simulink model "V2GStronge2_published_controller"  (R2024a)
settings: Solver=odeN  StartTime=0.0  StopTime=36000  FixedStep=10
model workspace (MAT data in the model file):
  Soc = 75
undefined symbols (not defined in the file): Ion, Lithium
libraries: spsMosfetLib x14, spsSeriesRLCBranchLib x14, slpidlib x8, spsBatteryLib x4, spsPWMGeneratorDCDCLib x4, spsCurrentMeasurementLib x3, spsAlphaBetaZerotodq0Lib x2, spsGroundLib x1, spsPWMGenerator2LevelLib x1, eePowerMeasurement x1, spsThreePhaseVIMeasurementLib x1, spsThreePhaseSourceLib x1
(part 1 of 2)
settings Model: SimulationMode=accelerator  PacingRate=1000  VariantFading=off  Creator=Mahmoud Kiasari  LastModifiedBy=mtk17
settings SolverCC: ZeroCrossControl=DisableAll  ZeroCrossAlgorithm=Adaptive  ODENIntegrationMethod=ode1
settings DataIOCC: ExternalInput=HouseHoldConsumption  SaveOutput=off  SignalLogging=off  DSMLogging=off  SaveTime=off  ReturnWorkspaceOutputs=off  OutputOption=SpecifiedOutputTimes  OutputTimes=OutTime
settings OptimizationCC: DefaultUnderspecifiedDataType=single  ReuseModelBlockBuffer=off
settings DebuggingCC: IgnoredZcDiagnostic=none  UnconnectedInputMsg=warning  UnconnectedOutputMsg=warning  UnconnectedLineMsg=warning
settings ModelReferenceCC: UpdateModelReferenceTargets=AssumeUpToDate  CheckModelReferenceTargetMessage=warning  EnableParallelModelReferenceBuilds=on  ModelReferenceNumInstancesAllowed=Zero  PropagateSignalLabelsOutOfModel=off
settings SFSimCC: SimTargetLang=C++  GPUAcceleration=on  SimDLTargetLibrary=cudnn
settings RTWCC: GPUComputeCapability=3.5  DLArmComputeVersion=19.05

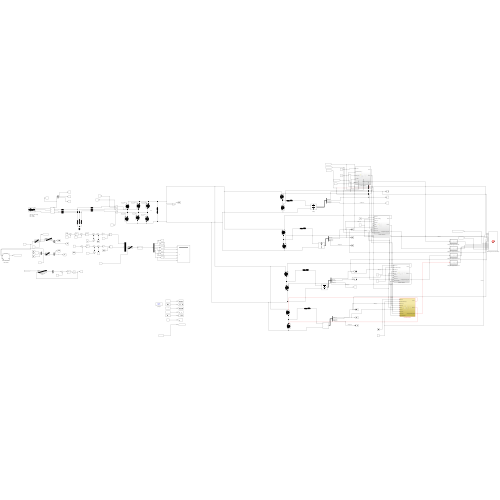
[thumbnail: Simulink's stored preview of the top-level diagram]
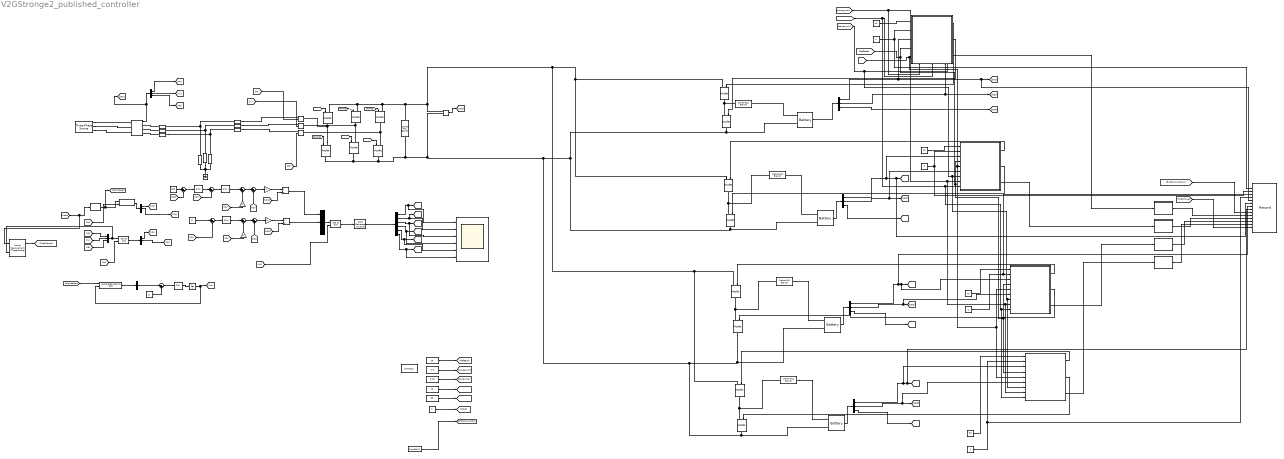
== system V2GStronge2_published_controller ==
  note: Battery
  note: Vdc
  note: 208V line to line voltage
      | Fsw = 10Khz
      | Fres = 1000hz
  Alpha-Beta-Zero to dq0 : spsAlphaBetaZerotodq0Lib/Alpha-Beta-Zero to dq0  Alignment=90 degrees behind phase A axis
  Alpha-Beta-Zero to dq1 : spsAlphaBetaZerotodq0Lib/Alpha-Beta-Zero to dq0  Alignment=90 degrees behind phase A axis
  Battery : spsBatteryLib/Battery  BatType=Lithium-Ion  ShowTempParam=off  ThermalPreset=no  ShowAgeParam=off  NomV=360  NomQ=62  SOC=90  Batt_Tr=1  PresetModel=off  MaxQ=300  MinV=270  FullV=419.0354  Dis_rate=130.4348  R=0.012  Normal_OP=271.3043  expZone="[388.9389      14.73913]"  current=[6.5 13 32.5]  Units=Time  Tci=20  NomT=20  T2=0  MaxQ2=300  FullV2=300  Normal_OP2=270  expZone2="[388.9389      14.73913]"  Rca=0.6411  ti=4880  Dp=0  Neq0=0  Tsim=1e6  Ta1=25  Qeol=5.4*0.9  Reol=0.013333*1.2  Char_age=[2.3478, 3]  Dis_age=[2.3478, 10]  N1=1500  N2=10500  N3=1000  N4=1400  Ta2=45  N5=950
  Battery1 : spsBatteryLib/Battery  BatType=Lithium-Ion  ShowTempParam=off  ThermalPreset=no  ShowAgeParam=off  NomV=375  NomQ=100  SOC=70  Batt_Tr=1  PresetModel=on  MaxQ=100  MinV=281.25  FullV=436.4952  Dis_rate=43.4783  R=0.0375  Normal_OP=90.4348  expZone="[405.1447      4.913043]"  current=[6.5 13 32.5]  Units=Time  Tci=20  NomT=20  T2=0  MaxQ2=300  FullV2=300  Normal_OP2=270  expZone2="[388.9389      14.73913]"  Rca=0.6411  ti=4880  Dp=0  Neq0=0  Tsim=1e6  Ta1=25  Qeol=5.4*0.9  Reol=0.013333*1.2  Char_age=[2.3478, 3]  Dis_age=[2.3478, 10]  N1=1500  N2=10500  N3=1000  N4=1400  Ta2=45  N5=950
  Battery2 : spsBatteryLib/Battery  BatType=Lithium-Ion  ShowTempParam=off  ThermalPreset=no  ShowAgeParam=off  NomV=360  NomQ=94  SOC=50  Batt_Tr=1  PresetModel=off  MaxQ=300  MinV=270  FullV=419.0354  Dis_rate=130.4348  R=0.012  Normal_OP=271.3043  expZone="[388.9389      14.73913]"  current=[6.5 13 32.5]  Units=Ampere-hour  Tci=20  NomT=20  T2=0  MaxQ2=300  FullV2=300  Normal_OP2=270  expZone2="[388.9389      14.73913]"  Rca=0.6411  ti=4880  Dp=0  Neq0=0  Tsim=1e6  Ta1=25  Qeol=5.4*0.9  Reol=0.013333*1.2  Char_age=[2.3478, 3]  Dis_age=[2.3478, 10]  N1=1500  N2=10500  N3=1000  N4=1400  Ta2=45  N5=950
  Battery3 : spsBatteryLib/Battery  BatType=Lithium-Ion  ShowTempParam=off  ThermalPreset=no  ShowAgeParam=off  NomV=396  NomQ=95  SOC=30  Batt_Tr=1  PresetModel=on  MaxQ=95  MinV=297  FullV=460.9389  Dis_rate=41.3043  R=0.041684  Normal_OP=85.913  expZone="[427.8328      4.667391]"  current=[6.5 13 32.5]  Units=Time  Tci=20  NomT=20  T2=0  MaxQ2=300  FullV2=300  Normal_OP2=270  expZone2="[388.9389      14.73913]"  Rca=0.6411  ti=4880  Dp=0  Neq0=0  Tsim=1e6  Ta1=25  Qeol=5.4*0.9  Reol=0.013333*1.2  Char_age=[2.3478, 3]  Dis_age=[2.3478, 10]  N1=1500  N2=10500  N3=1000  N4=1400  Ta2=45  N5=950
  Bus Selector{,1..3} (4 alike) : BusSelector  OutputSignals=SOC (%),Current (A),Voltage (V)
  Charge/Discharge/Ideal Detection : Subsystem  TreatAsAtomicUnit=on
  Charge/Discharge/Ideal Detection1 : Subsystem  TreatAsAtomicUnit=on
  Charge/Discharge/Ideal Detection2 : Subsystem  TreatAsAtomicUnit=on
  Charge/Discharge/Ideal Detection3 : Subsystem  TreatAsAtomicUnit=on
  Condition checker 1 : Subsystem
      settings: PortSchema="{\"entries\":[{\"content\":{\"sides\":[{\"content\":{\"connectorIds\":[\"In1\",\"In2\",\"In3\",\"In4\",\"In5\"]},\"type\":\"ConnectorPlacement.EquallySpacedRectSide\",\"uuid\":\"c002707d-8367-4a40-a9c2-601c499a357e\"},{\"content\":{\"connectorIds\":[\"Out1\",\"Out2\",\"Out3\"],\"side\":\"RIGHT\"},\"type\":\"ConnectorPlacement.EquallySpacedRectSide\",\"uuid\":\"668af4fe-86d6-4dea-905e-b454fc1f82cc\"},{\"content\":{\"side\":\"TOP\"},\"type\":\"ConnectorPlacement.EquallySpacedRectSide\",\"uuid\":\"2ab59da3-7144-4706-b30d-a458153a4ce4\"},{\"content\":{\"connectorIds\":[\"In6\",\"In7\",\"In8\"],\"side\":\"BOTTOM\"},\"type\":\"ConnectorPlacement.EquallySpacedRectSide\",\"uuid\":\"16d703a8-fda5-4631-9c2f-f2e45db3531f\"}]},\"type\":\"ConnectorPlacement.EquallySpacedConnector\",\"uuid\":\"736966d1-dbcb-4619-a26f-9e7ed5309763\"}],\"packageUris\":[\"http://schema.mathworks.com/mf0/Connector/R2020b\"],\"version\":\"1.0\"}"
  Condition checker 2 : Subsystem
  Condition checker 3 : Subsystem
  Condition checker 4 : Subsystem
  Constant : Constant  Value=0
  Constant1 : Constant  Value=400
  Constant10 : Constant  SampleTime=0
  Constant{6,9,12..13} (4 alike) : Constant  Value=40  SampleTime=0
  Constant14 : Constant  Value=-1  SampleTime=0
  Constant15 : Constant  Value=50  SampleTime=0
  Constant16 : Constant  SampleTime=0
  Constant17 : Constant  SampleTime=0
  Constant2 : Constant  Value=0
  Constant3 : Constant  Value=20  SampleTime=0
  Constant4 : Constant  Value=2.9  SampleTime=0
  Constant5 : Constant  Value=9.25  SampleTime=0
  Constant7 : Constant  Value=60  SampleTime=0
  Constant8 : Constant  Value=0  SampleTime=0
  Current Measurement : spsCurrentMeasurementLib/Current Measurement  PhasorSimulation=off  OutputType=Complex  PSBequivalent=0
  Current Measurement1 : spsCurrentMeasurementLib/Current Measurement  PhasorSimulation=off  OutputType=Complex  PSBequivalent=0
  Current Measurement2 : spsCurrentMeasurementLib/Current Measurement  PhasorSimulation=off  OutputType=Complex  PSBequivalent=0
  Demux{,1..2,4} (4 alike) : Demux  Outputs=3
  Demux3 : Demux  Outputs=6
  From Workspace : FromWorkspace  VariableName=from3to12  SampleTime=60
  Gain : Gain  Gain=2*3.14*60*10e-3
  Gain1 : Gain  Gain=2
  Gain2 : Gain  Gain=2*3.14*60*10e-3
  Gain3 : Gain  Gain=2
  Ground2 : spsGroundLib/Ground  LConnTagsString=a
  Integrator : Integrator
  Mosfet{,1,3..14} (14 alike) : spsMosfetLib/Mosfet  Ron=0.1  Lon=0  Rd=0.01  Vfd=0  IC=0  Rs=1e5  Cs=inf  Measurements=off
  Mux : Mux  Inputs=3
  Mux1 : Mux  Inputs=3
  PID Controller : slpidlib/PID Controller  Controller=PI  Form=Parallel  TimeDomain=Discrete-time  UseExternalTs=off  SampleTime=-1  IntegratorMethod=Forward Euler  FilterMethod=Forward Euler  ControllerParametersSource=internal  P=10  I=50000  UseKiTs=off  D=0  UseExternalDerivativeSource=off  N=100  UseFilter=on  TunerSelectOption=Transfer Function Based (PID Tuner App)  InitialConditionSource=internal  InitialConditionForIntegrator=0  InitialConditionForFilter=0  DifferentiatorICPrevScaledInput=0  ExternalReset=none  TrackingMode=off  Kt=1  LimitOutput=off  SatLimitsSource=internal  UpperSaturationLimit=0.95  LowerSaturationLimit=0  LinearizeAsGain=on  AntiWindupMode=none  Kb=1  LimitIntegrator=off  UpperIntegratorSaturationLimit=inf  LowerIntegratorSaturationLimit=-inf  POutMin=[]  POutMax=[]  IOutMin=[]  IOutMax=[]  DOutMin=[]  DOutMax=[]  NOutMin=[]  NOutMax=[]  SumOutMin=[]  SumOutMax=[]  SaturationOutMin=[]  SaturationOutMax=[]  PParamMin=[]  PParamMax=[]  IParamMin=[]  IParamMax=[]  DParamMin=[]  DParamMax=[]  NParamMin=[]  NParamMax=[]  KbParamMin=[]  KbParamMax=[]  KtParamMin=[]  KtParamMax=[]  KbOutMin=[]  KbOutMax=[]  KtOutMin=[]  KtOutMax=[]  IntegratorOutMin=[]  IntegratorOutMax=[]  FilterOutMin=[]  FilterOutMax=[]  SumI1OutMin=[]  SumI1OutMax=[]  SumI2OutMin=[]  SumI2OutMax=[]  SumI3OutMin=[]  SumI3OutMax=[]  SumI4OutMin=[]  SumI4OutMax=[]  SumDOutMin=[]  SumDOutMax=[]  DifferentiatorOutMin=[]  DifferentiatorOutMax=[]  FilterDiffOutCoefMin=[]  FilterDiffOutCoefMax=[]  ReciprocalOutMin=[]  ReciprocalOutMax=[]  SumDenOutMin=[]  SumDenOutMax=[]  SumNumOutMin=[]  SumNumOutMax=[]  DivideOutMin=[]  DivideOutMax=[]  UdiffTsProdOutMin=[]  UdiffTsProdOutMax=[]  NTsProdOutMin=[]  NTsProdOutMax=[]  UintegralTsProdOutMin=[]  UintegralTsProdOutMax=[]  UngainTsProdOutMin=[]  UngainTsProdOutMax=[]  ClampingZeroOutDataTypeStr=Inherit: Inherit via back propagation  ClampingZeroOutMin=[]  ClampingZeroOutMax=[]  FilterDenConstantOutDataTypeStr=Inherit: Inherit via back propagation  FilterDenConstantOutMin=[]  FilterDenConstantOutMax=[]  PCopyOutDataTypeStr=Inherit: Inherit via back propagation  PCopyOutMin=[]  PCopyOutMax=[]  NCopyOutDataTypeStr=Inherit: Inherit via back propagation  NCopyOutMin=[]  NCopyOutMax=[]  IntegratorContinuousStateAttributes=''  IntegratorStateMustResolveToSignalObject=off  IntegratorRTWStateStorageClass=Auto  FilterContinuousStateAttributes=''  FilterStateMustResolveToSignalObject=off  FilterRTWStateStorageClass=Auto  ParallelPVariant=InternalParameters  IdealPVariant=Disabled  IVariant=InternalParameters  DVariant=Disabled  IntegratorVariant=Discrete  SatVariant=Disabled  AWVariant=Passthrough  PCopyVariant=Disabled  TRVariant=Disabled  FdbkBlocksVariant=Forward  IdealPFdbkVariant=Disabled  SatFdbkVariant=Disabled  DerivativeFilterVariant=Disabled  NVariant=Disabled  NCopyVariant=Disabled_SignalSpec  FilterICVariant=Disabled  IntegratorICVariant=InternalICs  ExternalResetVariant=Disabled  TRSumVariant=Passthrough  SumFdbkVariant=Disabled  SumVariant=Sum_PI  TsampFilterVariant=InternalTs  TsampNgainVariant=Passthrough  TsampIntegralVariant=Disabled_SignalSpec  ExternalSaturationOutDataTypeStr=Inherit: Same as second input  DerivativeSourceVariant=Disabled
  PID Controller1 : slpidlib/PID Controller  Controller=PI  Form=Parallel  TimeDomain=Continuous-time  UseExternalTs=off  SampleTime=-1  IntegratorMethod=Forward Euler  FilterMethod=Forward Euler  ControllerParametersSource=internal  P=0.5  I=5  UseKiTs=off  D=0  UseExternalDerivativeSource=off  N=100  UseFilter=on  TunerSelectOption=Transfer Function Based (PID Tuner App)  InitialConditionSource=internal  InitialConditionForIntegrator=0  InitialConditionForFilter=0  DifferentiatorICPrevScaledInput=0  ExternalReset=none  TrackingMode=off  Kt=1  LimitOutput=off  SatLimitsSource=internal  UpperSaturationLimit=inf  LowerSaturationLimit=-inf  LinearizeAsGain=on  AntiWindupMode=none  Kb=1  LimitIntegrator=off  UpperIntegratorSaturationLimit=inf  LowerIntegratorSaturationLimit=-inf  POutMin=[]  POutMax=[]  IOutMin=[]  IOutMax=[]  DOutMin=[]  DOutMax=[]  NOutMin=[]  NOutMax=[]  SumOutMin=[]  SumOutMax=[]  SaturationOutMin=[]  SaturationOutMax=[]  PParamMin=[]  PParamMax=[]  IParamMin=[]  IParamMax=[]  DParamMin=[]  DParamMax=[]  NParamMin=[]  NParamMax=[]  KbParamMin=[]  KbParamMax=[]  KtParamMin=[]  KtParamMax=[]  KbOutMin=[]  KbOutMax=[]  KtOutMin=[]  KtOutMax=[]  IntegratorOutMin=[]  IntegratorOutMax=[]  FilterOutMin=[]  FilterOutMax=[]  SumI1OutMin=[]  SumI1OutMax=[]  SumI2OutMin=[]  SumI2OutMax=[]  SumI3OutMin=[]  SumI3OutMax=[]  SumI4OutMin=[]  SumI4OutMax=[]  SumDOutMin=[]  SumDOutMax=[]  DifferentiatorOutMin=[]  DifferentiatorOutMax=[]  FilterDiffOutCoefMin=[]  FilterDiffOutCoefMax=[]  ReciprocalOutMin=[]  ReciprocalOutMax=[]  SumDenOutMin=[]  SumDenOutMax=[]  SumNumOutMin=[]  SumNumOutMax=[]  DivideOutMin=[]  DivideOutMax=[]  UdiffTsProdOutMin=[]  UdiffTsProdOutMax=[]  NTsProdOutMin=[]  NTsProdOutMax=[]  UintegralTsProdOutMin=[]  UintegralTsProdOutMax=[]  UngainTsProdOutMin=[]  UngainTsProdOutMax=[]  ClampingZeroOutDataTypeStr=Inherit: Inherit via back propagation  ClampingZeroOutMin=[]  ClampingZeroOutMax=[]  FilterDenConstantOutDataTypeStr=Inherit: Inherit via back propagation  FilterDenConstantOutMin=[]  FilterDenConstantOutMax=[]  PCopyOutDataTypeStr=Inherit: Inherit via back propagation  PCopyOutMin=[]  PCopyOutMax=[]  NCopyOutDataTypeStr=Inherit: Inherit via back propagation  NCopyOutMin=[]  NCopyOutMax=[]  IntegratorContinuousStateAttributes=''  IntegratorStateMustResolveToSignalObject=off  IntegratorRTWStateStorageClass=Auto  FilterContinuousStateAttributes=''  FilterStateMustResolveToSignalObject=off  FilterRTWStateStorageClass=Auto  ParallelPVariant=InternalParameters  IdealPVariant=Disabled  IVariant=InternalParameters  DVariant=Disabled  IntegratorVariant=Continuous  SatVariant=Disabled  AWVariant=Passthrough  PCopyVariant=Disabled  TRVariant=Disabled  FdbkBlocksVariant=Forward  IdealPFdbkVariant=Disabled  SatFdbkVariant=Disabled  DerivativeFilterVariant=Disabled  NVariant=Disabled  NCopyVariant=Disabled_SignalSpec  FilterICVariant=Disabled  IntegratorICVariant=InternalICs  ExternalResetVariant=Disabled  TRSumVariant=Passthrough  SumFdbkVariant=Disabled  SumVariant=Sum_PI  TsampFilterVariant=InternalTs  TsampNgainVariant=Passthrough  TsampIntegralVariant=Disabled_SignalSpec  ExternalSaturationOutDataTypeStr=Inherit: Same as second input  DerivativeSourceVariant=Disabled
  PID Controller2 : slpidlib/PID Controller  Controller=PI  Form=Parallel  TimeDomain=Continuous-time  UseExternalTs=off  SampleTime=-1  IntegratorMethod=Forward Euler  FilterMethod=Forward Euler  ControllerParametersSource=internal  P=25  I=500  UseKiTs=off  D=0  UseExternalDerivativeSource=off  N=100  UseFilter=on  TunerSelectOption=Transfer Function Based (PID Tuner App)  InitialConditionSource=internal  InitialConditionForIntegrator=0  InitialConditionForFilter=0  DifferentiatorICPrevScaledInput=0  ExternalReset=none  TrackingMode=off  Kt=1  LimitOutput=off  SatLimitsSource=internal  UpperSaturationLimit=inf  LowerSaturationLimit=-inf  LinearizeAsGain=on  AntiWindupMode=none  Kb=1  LimitIntegrator=off  UpperIntegratorSaturationLimit=inf  LowerIntegratorSaturationLimit=-inf  POutMin=[]  POutMax=[]  IOutMin=[]  IOutMax=[]  DOutMin=[]  DOutMax=[]  NOutMin=[]  NOutMax=[]  SumOutMin=[]  SumOutMax=[]  SaturationOutMin=[]  SaturationOutMax=[]  PParamMin=[]  PParamMax=[]  IParamMin=[]  IParamMax=[]  DParamMin=[]  DParamMax=[]  NParamMin=[]  NParamMax=[]  KbParamMin=[]  KbParamMax=[]  KtParamMin=[]  KtParamMax=[]  KbOutMin=[]  KbOutMax=[]  KtOutMin=[]  KtOutMax=[]  IntegratorOutMin=[]  IntegratorOutMax=[]  FilterOutMin=[]  FilterOutMax=[]  SumI1OutMin=[]  SumI1OutMax=[]  SumI2OutMin=[]  SumI2OutMax=[]  SumI3OutMin=[]  SumI3OutMax=[]  SumI4OutMin=[]  SumI4OutMax=[]  SumDOutMin=[]  SumDOutMax=[]  DifferentiatorOutMin=[]  DifferentiatorOutMax=[]  FilterDiffOutCoefMin=[]  FilterDiffOutCoefMax=[]  ReciprocalOutMin=[]  ReciprocalOutMax=[]  SumDenOutMin=[]  SumDenOutMax=[]  SumNumOutMin=[]  SumNumOutMax=[]  DivideOutMin=[]  DivideOutMax=[]  UdiffTsProdOutMin=[]  UdiffTsProdOutMax=[]  NTsProdOutMin=[]  NTsProdOutMax=[]  UintegralTsProdOutMin=[]  UintegralTsProdOutMax=[]  UngainTsProdOutMin=[]  UngainTsProdOutMax=[]  ClampingZeroOutDataTypeStr=Inherit: Inherit via back propagation  ClampingZeroOutMin=[]  ClampingZeroOutMax=[]  FilterDenConstantOutDataTypeStr=Inherit: Inherit via back propagation  FilterDenConstantOutMin=[]  FilterDenConstantOutMax=[]  PCopyOutDataTypeStr=Inherit: Inherit via back propagation  PCopyOutMin=[]  PCopyOutMax=[]  NCopyOutDataTypeStr=Inherit: Inherit via back propagation  NCopyOutMin=[]  NCopyOutMax=[]  IntegratorContinuousStateAttributes=''  IntegratorStateMustResolveToSignalObject=off  IntegratorRTWStateStorageClass=Auto  FilterContinuousStateAttributes=''  FilterStateMustResolveToSignalObject=off  FilterRTWStateStorageClass=Auto  ParallelPVariant=InternalParameters  IdealPVariant=Disabled  IVariant=InternalParameters  DVariant=Disabled  IntegratorVariant=Continuous  SatVariant=Disabled  AWVariant=Passthrough  PCopyVariant=Disabled  TRVariant=Disabled  FdbkBlocksVariant=Forward  IdealPFdbkVariant=Disabled  SatFdbkVariant=Disabled  DerivativeFilterVariant=Disabled  NVariant=Disabled  NCopyVariant=Disabled_SignalSpec  FilterICVariant=Disabled  IntegratorICVariant=InternalICs  ExternalResetVariant=Disabled  TRSumVariant=Passthrough  SumFdbkVariant=Disabled  SumVariant=Sum_PI  TsampFilterVariant=InternalTs  TsampNgainVariant=Passthrough  TsampIntegralVariant=Disabled_SignalSpec  ExternalSaturationOutDataTypeStr=Inherit: Same as second input  DerivativeSourceVariant=Disabled
  PID Controller3 : slpidlib/PID Controller  Controller=PI  Form=Parallel  TimeDomain=Continuous-time  UseExternalTs=off  SampleTime=-1  IntegratorMethod=Forward Euler  FilterMethod=Forward Euler  ControllerParametersSource=internal  P=25  I=500  UseKiTs=off  D=0  UseExternalDerivativeSource=off  N=100  UseFilter=on  TunerSelectOption=Transfer Function Based (PID Tuner App)  InitialConditionSource=internal  InitialConditionForIntegrator=0  InitialConditionForFilter=0  DifferentiatorICPrevScaledInput=0  ExternalReset=none  TrackingMode=off  Kt=1  LimitOutput=off  SatLimitsSource=internal  UpperSaturationLimit=inf  LowerSaturationLimit=-inf  LinearizeAsGain=on  AntiWindupMode=none  Kb=1  LimitIntegrator=off  UpperIntegratorSaturationLimit=inf  LowerIntegratorSaturationLimit=-inf  POutMin=[]  POutMax=[]  IOutMin=[]  IOutMax=[]  DOutMin=[]  DOutMax=[]  NOutMin=[]  NOutMax=[]  SumOutMin=[]  SumOutMax=[]  SaturationOutMin=[]  SaturationOutMax=[]  PParamMin=[]  PParamMax=[]  IParamMin=[]  IParamMax=[]  DParamMin=[]  DParamMax=[]  NParamMin=[]  NParamMax=[]  KbParamMin=[]  KbParamMax=[]  KtParamMin=[]  KtParamMax=[]  KbOutMin=[]  KbOutMax=[]  KtOutMin=[]  KtOutMax=[]  IntegratorOutMin=[]  IntegratorOutMax=[]  FilterOutMin=[]  FilterOutMax=[]  SumI1OutMin=[]  SumI1OutMax=[]  SumI2OutMin=[]  SumI2OutMax=[]  SumI3OutMin=[]  SumI3OutMax=[]  SumI4OutMin=[]  SumI4OutMax=[]  SumDOutMin=[]  SumDOutMax=[]  DifferentiatorOutMin=[]  DifferentiatorOutMax=[]  FilterDiffOutCoefMin=[]  FilterDiffOutCoefMax=[]  ReciprocalOutMin=[]  ReciprocalOutMax=[]  SumDenOutMin=[]  SumDenOutMax=[]  SumNumOutMin=[]  SumNumOutMax=[]  DivideOutMin=[]  DivideOutMax=[]  UdiffTsProdOutMin=[]  UdiffTsProdOutMax=[]  NTsProdOutMin=[]  NTsProdOutMax=[]  UintegralTsProdOutMin=[]  UintegralTsProdOutMax=[]  UngainTsProdOutMin=[]  UngainTsProdOutMax=[]  ClampingZeroOutDataTypeStr=Inherit: Inherit via back propagation  ClampingZeroOutMin=[]  ClampingZeroOutMax=[]  FilterDenConstantOutDataTypeStr=Inherit: Inherit via back propagation  FilterDenConstantOutMin=[]  FilterDenConstantOutMax=[]  PCopyOutDataTypeStr=Inherit: Inherit via back propagation  PCopyOutMin=[]  PCopyOutMax=[]  NCopyOutDataTypeStr=Inherit: Inherit via back propagation  NCopyOutMin=[]  NCopyOutMax=[]  IntegratorContinuousStateAttributes=''  IntegratorStateMustResolveToSignalObject=off  IntegratorRTWStateStorageClass=Auto  FilterContinuousStateAttributes=''  FilterStateMustResolveToSignalObject=off  FilterRTWStateStorageClass=Auto  ParallelPVariant=InternalParameters  IdealPVariant=Disabled  IVariant=InternalParameters  DVariant=Disabled  IntegratorVariant=Continuous  SatVariant=Disabled  AWVariant=Passthrough  PCopyVariant=Disabled  TRVariant=Disabled  FdbkBlocksVariant=Forward  IdealPFdbkVariant=Disabled  SatFdbkVariant=Disabled  DerivativeFilterVariant=Disabled  NVariant=Disabled  NCopyVariant=Disabled_SignalSpec  FilterICVariant=Disabled  IntegratorICVariant=InternalICs  ExternalResetVariant=Disabled  TRSumVariant=Passthrough  SumFdbkVariant=Disabled  SumVariant=Sum_PI  TsampFilterVariant=InternalTs  TsampNgainVariant=Passthrough  TsampIntegralVariant=Disabled_SignalSpec  ExternalSaturationOutDataTypeStr=Inherit: Same as second input  DerivativeSourceVariant=Disabled
  PWM Generator (2-Level) : spsPWMGenerator2LevelLib/PWM Generator (2-Level)  ModulatorType=Three-phase bridge (6 pulses)  ModulatorMode=Unsynchronized  Fc=60  Pc=90  nF=27  MinMax="[ -1  1 ]"  SamplingTechnique=Natural  ModulatingSignals=off  m=0.8  Freq=60  Phase=0  Ts=0  ShowCarrierOutport=off
  Power Measurement (Three-Phase) : eePowerMeasurement/Power Measurement (Three-Phase)  LabelModeActiveChoice=Continuous  F=60  K=[0 1 2 3]  Seq=Positive  Ts=0
  Product : Product  Inputs=*/
  Product1 : Product  Inputs=*/
  Recording the SoC of each battery : Record  Filename=C:\Users\Mahmoud Kiasari\Desktop\Dalhousie\Thesis\Thesis Versions\Matlab Models\EV V2G and G2V\Data\ThesisData2Hours12to6.xlsx  FileSettingsInternal="{\"entries\":[{\"content\":{\"excelSettings\":{\"content\":{},\"type\":\"Streamout.ExcelSettings\"}},\"type\":\"Streamout.FileSettingStorage\",\"uuid\":\"\"}],\"packageUris\":[\"http:\\/\\/schema.mathworks.com\\/mf0\\/streamout_blocks\\/R2020a\"],\"version\":\"1.0\"}"  Layout=[1 1]  SignalsInternal="{\"entries\":[{\"content\":{\"signals\":[{\"content\":{\"blockPath\":[],\"dimensions\":[1],\"domain\":\"\",\"lineColor\":\"#64d413\",\"port\":1,\"sid\":[\"\"],\"signalID\":1,\"signalName\":\"Owner 1\"},\"type\":\"RecordBlkView.Signal\",\"uuid\":\"\"},{\"content\":{\"blockPath\":[],\"dimensions\":[1],\"domain\":\"\",\"lineColor\":\"#64d413\",\"plots\":[ 9 ],\"port\":2,\"sid\":[\"\"],\"signalID\":2,\"signalName\":\"Owner 2\"},\"type\":\"RecordBlkView.Signal\",\"uuid\":\"\"},{\"content\":{\"blockPath\":[],\"dimensions\":[1],\"domain\":\"\",\"lineColor\":\"#ff13a6\",\"plots\":[ 2 ],\"port\":3,\"sid\":[\"\"],\"signalID\":3,\"signalName\":\"Owner 3\"},\"type\":\"RecordBlkView.Signal\",\"uuid\":\"\"},{\"content\":{\"blockPath\":[],\"dimensions\":[1],\"domain\":\"\",\"lineColor\":\"#fe330a\",\"plots\":[ 10 ],\"port\":4,\"sid\":[\"\"],\"signalID\":4,\"signalName\":\"Owner 4\"},\"type\":\"RecordBlkView.Signal\",\"uuid\":\"\"},{\"content\":{\"blockPath\":[],\"dimensions\":[1],\"domain\":\"\",\"lineColor\":\"#64d413\",\"port\":5,\"sid\":[\"\"],\"signalID\":5,\"signalName\":\"<SOC (%)>\"},\"type\":\"RecordBlkView.Signal\",\"uuid\":\"\"},{\"content\":{\"blockPath\":[],\"dimensions\":[1],\"domain\":\"\",\"lineColor\":\"#4dbeee\",\"port\":6,\"sid\":[\"\"],\"signalID\":6,\"signalName\":\"<SOC (%)>\"},\"type\":\"RecordBlkView.Signal\",\"uuid\":\"\"},{\"content\":{\"blockPath\":[],\"dimensions\":[1],\"domain\":\"\",\"lineColor\":\"#a2142f\",\"port\":7,\"sid\":[\"\"],\"signalID\":7,\"signalName\":\"<SOC (%)>\"},\"type\":\"RecordBlkView.Signal\",\"uuid\":\"\"},{\"content\":{\"blockPath\":[],\"dimensions\":[1],\"domain\":\"\",\"lineColor\":\"#139fff\",\"port\":8,\"sid\":[\"\"],\"signalID\":8,\"signalName\":\"<SOC (%)>\"},\"type\":\"RecordBlkView.Signal\",\"uuid\":\"\"},{\"content\":{\"blockPath\":[],\"dimensions\":[1],\"domain\":\"\",\"lineColor\":\"#ff6929\",\"plots\":[ 1 ],\"port\":9,\"sid\":[\"\"],\"signalID\":9,\"signalName\":\"From26\"},\"type\":\"RecordBlkView.Signal\",\"uuid\":\"\"},{\"content\":{\"blockPath\":[],\"dimensions\":[1],\"domain\":\"\",\"lineColor\":\"#a2142f\",\"port\":10,\"sid\":[\"\"],\"signalID\":10,\"signalName\":\"Charge\\/Discharge\\/Ideal Detection\"},\"type\":\"RecordBlkView.Signal\",\"uuid\":\"\"},{\"content\":{\"blockPath\":[],\"dimensions\":[1],\"domain\":\"\",\"lineColor\":\"#139fff\",\"port\":11,\"sid\":[\"\"],\"signalID\":11,\"signalName\":\"Charge\\/Discharge\\/Ideal Detection1\"},\"type\":\"RecordBlkView.Signal\",\"uuid\":\"\"},{\"content\":{\"blockPath\":[],\"dimensions\":[1],\"domain\":\"\",\"lineColor\":\"#ff6929\",\"port\":12,\"sid\":[\"\"],\"signalID\":12,\"signalName\":\"Charge\\/Discharge\\/Ideal Detection2\"},\"type\":\"RecordBlkView.Signal\",\"uuid\":\"\"},{\"content\":{\"blockPath\":[],\"dimensions\":[1],\"domain\":\"\",\"lineColor\":\"#b746ff\",\"port\":13,\"sid\":[\"\"],\"signalID\":13,\"signalName\":\"Charge\\/Discharge\\/Ideal Detection3\"},\"type\":\"RecordBlkView.Signal\",\"uuid\":\"\"},{\"content\":{\"blockPath\":[],\"dimensions\":[4],\"domain\":\"\",\"hasChildren\":true,\"lineColor\":\"#22b573\",\"lineWidth\":2,\"port\":14,\"sid\":[\"\"],\"signalID\":14,\"signalName\":\"From7\"},\"type\":\"RecordBlkView.Signal\",\"uuid\":\"\"},{\"content\":{\"blockPath\":[],\"channel\":[1],\"dimensions\":[4],\"domain\":\"\",\"lineColor\":\"#fe330a\",\"parentID\":14,\"port\":14,\"sid\":[\"\"],\"signalID\":15,\"signalName\":\"From7\"},\"type\":\"RecordBlkView.Signal\",\"uuid\":\"\"},{\"content\":{\"blockPath\":[],\"channel\":[2],\"dimensions\":[4],\"domain\":\"\",\"lineColor\":\"#fe330a\",\"parentID\":14,\"port\":14,\"sid\":[\"\"],\"signalID\":16,\"signalName\":\"From7\"},\"type\":\"RecordBlkView.Signal\",\"uuid\":\"\"},{\"content\":{\"blockPath\":[],\"channel\":[3],\"dimensions\":[4],\"domain\":\"\",\"lineColor\":\"#22b573\",\"parentID\":14,\"port\":14,\"sid\":[\"\"],\"signalID\":17,\"signalName\":\"From7\"},\"type\":\"RecordBlkView.Signal\",\"uuid\":\"\"},{\"content\":{\"blockPath\":[],\"channel\":[4],\"dimensions\":[4],\"domain\":\"\",\"lineColor\":\"#0072bd\",\"parentID\":14,\"port\":14,\"sid\":[\"\"],\"signalID\":18,\"signalName\":\"From7\"},\"type\":\"RecordBlkView.Signal\",\"uuid\":\"\"}]},\"type\":\"RecordBlkView.InputSignals\",\"uuid\":\"\"}],\"packageUris\":[\"http:\\/\\/schema.mathworks.com\\/mf0\\/streamout_blocks\\/R2020a\"],\"version\":\"1.0\"}"  VisualizationBindings="{\"sparklinesplugin\":{\"info\":[{\"bindingParametersList\":[],\"subplotID\":1}]}}"
  Scope1 : Scope  NumInputPorts=6
  Se : spsSeriesRLCBranchLib/Series RLC Branch  LConnTagsString=__new0  RConnTagsString=__new0  BranchType=RC  Resistance=1.31  Inductance=1e-3  SetiL0=off  InitialCurrent=0  Capacitance=156e-6  Setx0=off  InitialVoltage=0  Measurements=None
  Se1 : spsSeriesRLCBranchLib/Series RLC Branch  LConnTagsString=__new0  RConnTagsString=__new0  BranchType=RC  Resistance=1.31  Inductance=1e-3  SetiL0=off  InitialCurrent=0  Capacitance=156e-6  Setx0=off  InitialVoltage=0  Measurements=None
  Se2 : spsSeriesRLCBranchLib/Series RLC Branch  LConnTagsString=__new0  RConnTagsString=__new0  BranchType=RC  Resistance=1.31  Inductance=1e-3  SetiL0=off  InitialCurrent=0  Capacitance=156e-6  Setx0=off  InitialVoltage=0  Measurements=None
  Series RLC Branch1 : spsSeriesRLCBranchLib/Series RLC Branch  LConnTagsString=__new0  RConnTagsString=__new0  BranchType=RC  Resistance=1e-3  Inductance=1e-3  SetiL0=off  InitialCurrent=0  Capacitance=18e-3  Setx0=on  InitialVoltage=400  Measurements=None
  Series RLC Branch11 : spsSeriesRLCBranchLib/Series RLC Branch  LConnTagsString=__new0  RConnTagsString=__new0  BranchType=L  Resistance=1  Inductance=0.49e-3  SetiL0=off  InitialCurrent=0  Capacitance=1e-6  Setx0=off  InitialVoltage=0  Measurements=None
  Series RLC Branch{9,13,16..17} (4 alike) : spsSeriesRLCBranchLib/Series RLC Branch  LConnTagsString=__new0  RConnTagsString=__new0  BranchType=RL  Resistance=0.0001  Inductance=2e-3  SetiL0=off  InitialCurrent=0  Capacitance=1e-6  Setx0=off  InitialVoltage=0  Measurements=None
  Series RLC Branch2 : spsSeriesRLCBranchLib/Series RLC Branch  LConnTagsString=__new0  RConnTagsString=__new0  BranchType=L  Resistance=1  Inductance=0.69e-3  SetiL0=off  InitialCurrent=0  Capacitance=1e-6  Setx0=off  InitialVoltage=0  Measurements=None
  Series RLC Branch4 : spsSeriesRLCBranchLib/Series RLC Branch  LConnTagsString=__new0  RConnTagsString=__new0  BranchType=L  Resistance=1  Inductance=0.69e-3  SetiL0=off  InitialCurrent=0  Capacitance=1e-6  Setx0=off  InitialVoltage=0  Measurements=None
  Series RLC Branch5 : spsSeriesRLCBranchLib/Series RLC Branch  LConnTagsString=__new0  RConnTagsString=__new0  BranchType=L  Resistance=1  Inductance=0.69e-3  SetiL0=off  InitialCurrent=0  Capacitance=1e-6  Setx0=off  InitialVoltage=0  Measurements=None
  Series RLC Branch7 : spsSeriesRLCBranchLib/Series RLC Branch  LConnTagsString=__new0  RConnTagsString=__new0  BranchType=L  Resistance=1  Inductance=0.49e-3  SetiL0=off  InitialCurrent=0  Capacitance=1e-6  Setx0=off  InitialVoltage=0  Measurements=None
  Series RLC Branch8 : spsSeriesRLCBranchLib/Series RLC Branch  LConnTagsString=__new0  RConnTagsString=__new0  BranchType=L  Resistance=1  Inductance=0.49e-3  SetiL0=off  InitialCurrent=0  Capacitance=1e-6  Setx0=off  InitialVoltage=0  Measurements=None
  Sum : Sum  Inputs=|-+
  Sum{1..2,5..6} (4 alike) : Sum  Inputs=|+-
  Sum3 : Sum  Inputs=|++
  Sum4 : Sum  Inputs=|++
  Sum7 : Sum  Inputs=|++
  Three-Phase V-I Measurement1 : spsThreePhaseVIMeasurementLib/Three-Phase V-I Measurement  VoltageMeasurement=phase-to-ground  SetLabelV=off  LabelV=Vabc  Vpu=off  VpuLL=off  CurrentMeasurement=no  SetLabelI=off  LabelI=Iabc  Ipu=off  Pbase=100e6  Vbase=500e3  OutputType=Complex  PhasorSimulation=off  PSBequivalent=0
  Three-Phase Source : spsThreePhaseSourceLib/Three-Phase Source  InternalConnection=Yg  VoltagePhases=off  Voltage=480  PhaseAngle=0  Voltage_phases=[25e3 25e3 25e3]/sqrt(3)  PhaseAngles_phases=[0 -120 +120]  Frequency=60  NonIdealSource=on  SpecifyImpedance=off  Resistance=0.8929e-3  Inductance=16.58e-9  ShortCircuitLevel=100e6  BaseVoltage=480  XRratio=7  BusType=swing  Pref=10e3  Qref=0  Prefabc=[10e3, 10e3, 10e3]  Qrefabc=[0, 0, 0]  Qmin=-inf  Qmax=inf
  Voltage Measurement : spsVoltageMeasurementLib/Voltage Measurement  PhasorSimulation=off  OutputType=Complex  PSBequivalent=0
  abc to Alpha-Beta-Zero : spsabctoAlphaBetaZeroLib/abc to Alpha-Beta-Zero
  abc to dq0 : spsabctodq0Lib/abc to dq0  Alignment=90 degrees behind phase A axis
  dq0 to abc : spsdq0toabcLib/dq0 to abc  Alignment=90 degrees behind phase A axis
  powergui : spspowerguiLib/powergui  Priority=1  SimulationMode=Discrete  SampleTime=1e-4  frequency=60  Iterations=50  frequencyindice=0  Pbase=100e6  ErrMax=1e-4  UnitsV=kV  UnitsW=MW  buscounter=0  FunctionMessages=off  echomessages=off  EnableUseOfTLC=off  CurrentSourceSwitches=off  DisableSnubberDevices=off  DisableRonSwitches=off  DisableVfSwitches=off  DisplayEquations=off  AutomaticDiscreteSolvers=off  SolverType=Tustin/Backward Euler (TBE)  Interpol=off  ExternalGateDelay=off  methode=off  Ts=100  x0status=blocks  SPID=on  SwTol=0  HookPort=off  NonlinearTolerance=1e-4  nMaxIteration=100  ContinueOnMaxIteration=off  RestoreLinks=warning  ResistiveCurrentMeasurement=off  Frange=[0:2:500]  Ylog=off  Xlog=on  ShowGrid=off  save=off  variable=ZData  structure=0  ZoomFFT=off  StartTime=0.0  cycles=1  DisplayStyle=1  fundamental=60  FreqAxis=off  MaxFrequency=1000  frequencyindicesteady=1  RmsSteady=1  display=off
  wires:
  Current Measurement2/1 -> [IR]
  Current Measurement1/1 -> [IY]
  Current Measurement/1 -> [IB]
  Voltage Measurement/1 -> [VDC]
  Condition checker 1/1(Buck 1) -> Mosfet1/1
  Condition checker 1/2(Boost 1) -> Mosfet/1
  Bus Selector/1 -> Condition checker 1/3(<SOC (%)>), Recording the SoC of each battery/5, [SOC]  "<SOC (%)>"
  abc to Alpha-Beta-Zero/1 -> [alphabeta], Alpha-Beta-Zero to dq0/1
  Alpha-Beta-Zero to dq0/1 -> Demux/1
  Demux/2 -> [VQ]
  [IR] -> Mux/1
  [IY] -> Mux/2
  [IB] -> Mux/3
  Demux1/1 -> [ID]
  abc to dq0/1 -> Demux1/1
  Demux2/2 -> Sum/1
  [alphabeta] -> Alpha-Beta-Zero to dq1/1
  PID Controller/1 -> Integrator/1
  Sum/1 -> PID Controller/1
  Integrator/1 -> [wt], Alpha-Beta-Zero to dq1/2
  Constant1/1 -> Sum1/1
  [VDC] -> Sum1/2
  Sum1/1 -> PID Controller1/1
  PID Controller1/1 -> Sum2/1
  [ID] -> Sum2/2
  Sum2/1 -> PID Controller2/1
  PID Controller2/1 -> Sum3/1
  Gain/1 -> Sum3/2
  [IQ] -> Gain/1
  Sum3/1 -> Sum4/1
  [VD] -> Sum4/2
  Sum4/1 -> Gain1/1
  Gain1/1 -> Product/1
  [VDC] -> Product/2
  [VQ] -> Sum7/2
  Gain2/1 -> Sum6/2
  Sum7/1 -> Gain3/1
  [ID] -> Gain2/1
  Sum5/1 -> PID Controller3/1
  Constant2/1 -> Sum5/1
  [IQ] -> Sum5/2
  Gain3/1 -> Product1/1
  Sum6/1 -> Sum7/1
  [VDC] -> Product1/2
  PID Controller3/1 -> Sum6/1
  Product/1 -> Mux1/1
  Product1/1 -> Mux1/2
  Mux1/1 -> dq0 to abc/1
  dq0 to abc/1 -> PWM Generator (2-Level)/1
  PWM Generator (2-Level)/1 -> Demux3/1
  Demux3/1 -> Scope1/1, [PWM1]
  Demux3/2 -> Scope1/2, [PWM2]
  Demux3/3 -> Scope1/3, [PWM3]
  Demux3/4 -> Scope1/4, [PWM4]
  Demux3/5 -> Scope1/5, [PWM5]
  Demux3/6 -> Scope1/6, [PWM6]
  Demux1/2 -> [IQ]
  Three-Phase V-I Measurement1/1 -> [Vabc], Demux4/1
  Demux4/1 -> [VR]
  Demux4/2 -> [VY]
  Demux4/3 -> [VB]
  [wt] -> Alpha-Beta-Zero to dq0/2
  [wt] -> abc to dq0/2
  Demux/1 -> [VD]
  Alpha-Beta-Zero to dq1/1 -> Demux2/1
  [PWM1] -> Mosfet7/1
  [PWM3] -> Mosfet5/1
  [PWM5] -> Mosfet4/1
  [PWM2] -> Mosfet8/1
  [PWM4] -> Mosfet6/1
  [PWM6] -> Mosfet3/1
  Battery/1 -> Bus Selector/1
  Battery1/1 -> Bus Selector1/1
  Condition checker 2/2(Boost 2) -> Mosfet9/1
  Condition checker 2/1(Buck 2) -> Mosfet10/1
  Condition checker 4/2(Boost 4) -> Mosfet14/1
  Battery3/1 -> Bus Selector3/1
  Condition checker 4/1(Buck 4) -> Mosfet13/1
  Battery2/1 -> Bus Selector2/1
  Condition checker 3/2(Boost 3) -> Mosfet11/1
  Condition checker 3/1(Buck 3) -> Mosfet12/1
  Bus Selector2/2 -> Condition checker 3/6(Current), [Ibat2]  "<Current (A)>"
  Bus Selector2/3 -> [Vbat2]  "<Voltage (V)>"
  Constant3/1 -> [RefBase]
  Constant4/1 -> [power_min]
  Constant5/1 -> [power_max]
  Constant7/1 -> [bat_soc_max]
  Constant6/1 -> [bat_soc_min]
  From Workspace/1 -> [GridConsumption]
  Constant9/1 -> Condition checker 1/1(Min soc 1)
  Constant12/1 -> Condition checker 2/1(Min soc 2)
  Bus Selector1/1 -> Condition checker 2/3(<SOC (%)>), Recording the SoC of each battery/6, [SOC1]  "<SOC (%)>"
  Constant13/1 -> Condition checker 3/1(Min soc 3)
  Bus Selector2/1 -> Recording the SoC of each battery/7, Condition checker 3/3(<SOC (%)>), [SOC2]  "<SOC (%)>"
  Bus Selector3/1 -> Condition checker 4/3(<SOC (%)>), Recording the SoC of each battery/8, [SOC3]  "<SOC (%)>"
  Constant15/1 -> Condition checker 4/1(Min soc 4)
  [RefBase] -> Condition checker 2/4(Ref Base), Condition checker 4/4(Ref Base), Condition checker 3/4(Ref Base), Condition checker 1/4(Ref Base)
  [Clock] -> Condition checker 4/5(Clock), Condition checker 3/5(Clock), Condition checker 2/5(Clock), Condition checker 1/5(Clock)
  Charge/Discharge/Ideal Detection/1(Out1) -> Recording the SoC of each battery/10
  Charge/Discharge/Ideal Detection1/1(Out1) -> Recording the SoC of each battery/11
  Charge/Discharge/Ideal Detection2/1(Out1) -> Recording the SoC of each battery/12
  Charge/Discharge/Ideal Detection3/1(Out1) -> Recording the SoC of each battery/13
  [GridConsumption] -> Recording the SoC of each battery/9
  Constant17/1 -> [Clock]
  [power_max] -> Condition checker 4/8(power max), Condition checker 3/8(power max), Condition checker 2/8(power max), Condition checker 1/6(power max)
  [GridConsumption] -> Condition checker 4/9(grid consumption), Condition checker 3/9(grid consumption), Condition checker 2/9(grid consumption), Condition checker 1/7(grid consumption)
  [wt] -> dq0 to abc/2
  Constant10/1 -> Recording the SoC of each battery/1, Condition checker 1/2(ActiveDeactiveIdle_1)  "Owner 1"
  Constant8/1 -> Recording the SoC of each battery/2, Condition checker 2/2(ActiveDeactiveIdle_2)  "Owner 2"
  Constant14/1 -> Recording the SoC of each battery/3, Condition checker 3/2(ActiveDeactiveIdle_3)  "Owner 3"
  Constant16/1 -> Recording the SoC of each battery/4, Condition checker 4/2(ActiveDeactiveIdle_4)  "Owner 4"
  [power_min] -> Condition checker 4/7(power min), Condition checker 3/7(power min), Condition checker 2/7(power min)
  Condition checker 1/3(Charging Discharging Idle) -> Charge/Discharge/Ideal Detection/1(Input)
  Condition checker 2/3(Charging Discharging Idle) -> Charge/Discharge/Ideal Detection1/1(Input)
  Condition checker 3/3(Charging Discharging Idle) -> Charge/Discharge/Ideal Detection2/1(Input)
  Condition checker 4/3(Charging Discharging Idle) -> Charge/Discharge/Ideal Detection3/1(Input)
  Bus Selector/2 -> [Ibat], Condition checker 1/8(Current)  "<Current (A)>"
  Bus Selector/3 -> [Vbat]  "<Voltage (V)>"
  Constant/1 -> Sum/2
  Bus Selector1/3 -> [Vbat1]  "<Voltage (V)>"
  Bus Selector1/2 -> Condition checker 2/6(Current), [Ibat1]  "<Current (A)>"
  Bus Selector3/3 -> [Vbat3]  "<Voltage (V)>"
  Bus Selector3/2 -> Condition checker 4/6(Current), [Ibat3]  "<Current (A)>"
  Mux/1 -> Power Measurement (Three-Phase)/2, abc to dq0/1
  Power Measurement (Three-Phase)/1 -> [TotalPower]
  [Vabc] -> Power Measurement (Three-Phase)/1, abc to Alpha-Beta-Zero/1
  [TotalPower] -> Recording the SoC of each battery/14
  connections:
  Three-Phase Source/RConn2 -- Three-Phase V-I Measurement1/LConn2
  Three-Phase Source/RConn3 -- Three-Phase V-I Measurement1/LConn3
  Mosfet/LConn1 -- Series RLC Branch9/LConn1 -- Mosfet1/RConn1
  Three-Phase Source/RConn1 -- Three-Phase V-I Measurement1/LConn1
  Mosfet8/LConn1 -- Mosfet7/RConn1 -- Current Measurement2/LConn1
  Mosfet5/RConn1 -- Mosfet6/LConn1 -- Current Measurement1/LConn1
  Mosfet4/RConn1 -- Mosfet3/LConn1 -- Current Measurement/LConn1
  Battery/LConn1 -- Series RLC Branch9/RConn1
  Mosfet13/LConn1 -- Mosfet1/LConn1 -- Mosfet10/LConn1 -- Mosfet7/LConn1 -- Mosfet5/LConn1 -- Mosfet4/LConn1 -- Series RLC Branch1/LConn1 -- Voltage Measurement/LConn1 -- Mosfet12/LConn1
  Battery3/LConn2 -- Mosfet14/RConn1 -- Battery2/LConn2 -- Mosfet11/RConn1 -- Battery/LConn2 -- Mosfet/RConn1 -- Battery1/LConn2 -- Mosfet9/RConn1 -- Mosfet8/RConn1 -- Mosfet6/RConn1 -- Mosfet3/RConn1 -- Series RLC Branch1/RConn1 -- Voltage Measurement/LConn2
  Battery1/LConn1 -- Series RLC Branch13/RConn1
  Mosfet9/LConn1 -- Series RLC Branch13/LConn1 -- Mosfet10/RConn1
  Mosfet14/LConn1 -- Series RLC Branch16/LConn1 -- Mosfet13/RConn1
  Mosfet11/LConn1 -- Series RLC Branch17/LConn1 -- Mosfet12/RConn1
  Series RLC Branch16/RConn1 -- Battery3/LConn1
  Series RLC Branch17/RConn1 -- Battery2/LConn1
  Series RLC Branch5/RConn1 -- Series RLC Branch8/LConn1 -- Se/LConn1
  Series RLC Branch4/RConn1 -- Series RLC Branch7/LConn1 -- Se1/LConn1
  Se/RConn1 -- Ground2/LConn1 -- Se2/RConn1 -- Se1/RConn1
  Series RLC Branch11/LConn1 -- Series RLC Branch2/RConn1 -- Se2/LConn1
  Series RLC Branch11/RConn1 -- Current Measurement/RConn1
  Series RLC Branch8/RConn1 -- Current Measurement1/RConn1
  Series RLC Branch7/RConn1 -- Current Measurement2/RConn1
  Series RLC Branch4/LConn1 -- Three-Phase V-I Measurement1/RConn1
  Series RLC Branch5/LConn1 -- Three-Phase V-I Measurement1/RConn2
  Series RLC Branch2/LConn1 -- Three-Phase V-I Measurement1/RConn3

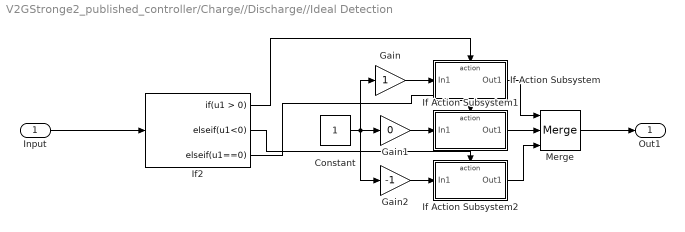
== system V2GStronge2_published_controller/Charge//Discharge//Ideal Detection ==
  Input : Inport
  Constant : Constant  SampleTime=0
  Gain : Gain
  Gain1 : Gain  Gain=0
  Gain2 : Gain  Gain=-1
  If Action Subsystem : Subsystem  TreatAsAtomicUnit=on
  If Action Subsystem1 : Subsystem  TreatAsAtomicUnit=on
  If Action Subsystem2 : Subsystem  TreatAsAtomicUnit=on
  If2 : If  ElseIfExpressions=u1<0, u1==0  ShowElse=off
  Merge : Merge  Inputs=3
  Out1 : Outport
  wires:
  Input/1 -> If2/1
  If2/2 -> If Action Subsystem2/Action
  If2/3 -> If Action Subsystem1/Action
  If2/1 -> If Action Subsystem/Action
  Gain/1 -> If Action Subsystem/1(In1)
  Constant/1 -> Gain2/1, Gain1/1, Gain/1
  Gain1/1 -> If Action Subsystem1/1(In1)
  Gain2/1 -> If Action Subsystem2/1(In1)
  If Action Subsystem/1(Out1) -> Merge/1
  If Action Subsystem1/1(Out1) -> Merge/2
  If Action Subsystem2/1(Out1) -> Merge/3
  Merge/1 -> Out1/1

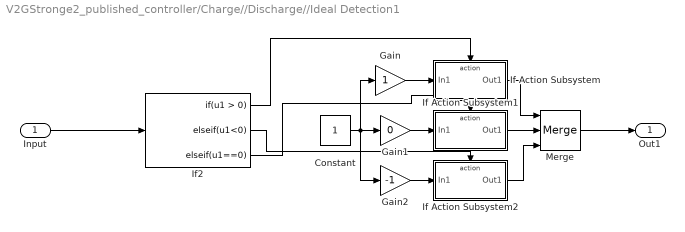
== system V2GStronge2_published_controller/Charge//Discharge//Ideal Detection1 ==
  Input : Inport
  Constant : Constant  SampleTime=0
  Gain : Gain
  Gain1 : Gain  Gain=0
  Gain2 : Gain  Gain=-1
  If Action Subsystem : Subsystem  TreatAsAtomicUnit=on
  If Action Subsystem1 : Subsystem  TreatAsAtomicUnit=on
  If Action Subsystem2 : Subsystem  TreatAsAtomicUnit=on
  If2 : If  ElseIfExpressions=u1<0, u1==0  ShowElse=off
  Merge : Merge  Inputs=3
  Out1 : Outport
  wires:
  Input/1 -> If2/1
  If2/2 -> If Action Subsystem2/Action
  If2/3 -> If Action Subsystem1/Action
  If2/1 -> If Action Subsystem/Action
  Gain/1 -> If Action Subsystem/1(In1)
  Constant/1 -> Gain2/1, Gain1/1, Gain/1
  Gain1/1 -> If Action Subsystem1/1(In1)
  Gain2/1 -> If Action Subsystem2/1(In1)
  If Action Subsystem/1(Out1) -> Merge/1
  If Action Subsystem1/1(Out1) -> Merge/2
  If Action Subsystem2/1(Out1) -> Merge/3
  Merge/1 -> Out1/1

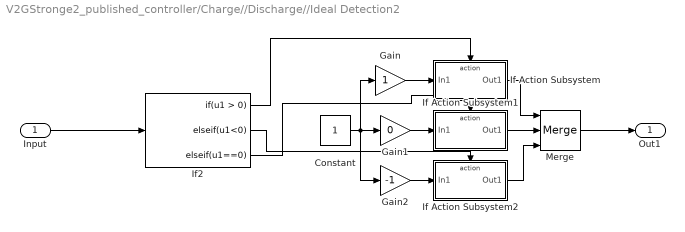
== system V2GStronge2_published_controller/Charge//Discharge//Ideal Detection2 ==
  Input : Inport
  Constant : Constant  SampleTime=0
  Gain : Gain
  Gain1 : Gain  Gain=0
  Gain2 : Gain  Gain=-1
  If Action Subsystem : Subsystem  TreatAsAtomicUnit=on
  If Action Subsystem1 : Subsystem  TreatAsAtomicUnit=on
  If Action Subsystem2 : Subsystem  TreatAsAtomicUnit=on
  If2 : If  ElseIfExpressions=u1<0, u1==0  ShowElse=off
  Merge : Merge  Inputs=3
  Out1 : Outport
  wires:
  Input/1 -> If2/1
  If2/2 -> If Action Subsystem2/Action
  If2/3 -> If Action Subsystem1/Action
  If2/1 -> If Action Subsystem/Action
  Gain/1 -> If Action Subsystem/1(In1)
  Constant/1 -> Gain2/1, Gain1/1, Gain/1
  Gain1/1 -> If Action Subsystem1/1(In1)
  Gain2/1 -> If Action Subsystem2/1(In1)
  If Action Subsystem/1(Out1) -> Merge/1
  If Action Subsystem1/1(Out1) -> Merge/2
  If Action Subsystem2/1(Out1) -> Merge/3
  Merge/1 -> Out1/1

== system V2GStronge2_published_controller/Charge//Discharge//Ideal Detection3 ==
  Input : Inport
  Constant : Constant  SampleTime=0
  Gain : Gain
  Gain1 : Gain  Gain=0
  Gain2 : Gain  Gain=-1
  If Action Subsystem : Subsystem  TreatAsAtomicUnit=on
  If Action Subsystem1 : Subsystem  TreatAsAtomicUnit=on
  If Action Subsystem2 : Subsystem  TreatAsAtomicUnit=on
  If2 : If  ElseIfExpressions=u1<0, u1==0  ShowElse=off
  Merge : Merge  Inputs=3
  Out1 : Outport
  wires:
  Input/1 -> If2/1
  If2/2 -> If Action Subsystem2/Action
  If2/3 -> If Action Subsystem1/Action
  If2/1 -> If Action Subsystem/Action
  Gain/1 -> If Action Subsystem/1(In1)
  Constant/1 -> Gain2/1, Gain1/1, Gain/1
  Gain1/1 -> If Action Subsystem1/1(In1)
  Gain2/1 -> If Action Subsystem2/1(In1)
  If Action Subsystem/1(Out1) -> Merge/1
  If Action Subsystem1/1(Out1) -> Merge/2
  If Action Subsystem2/1(Out1) -> Merge/3
  Merge/1 -> Out1/1

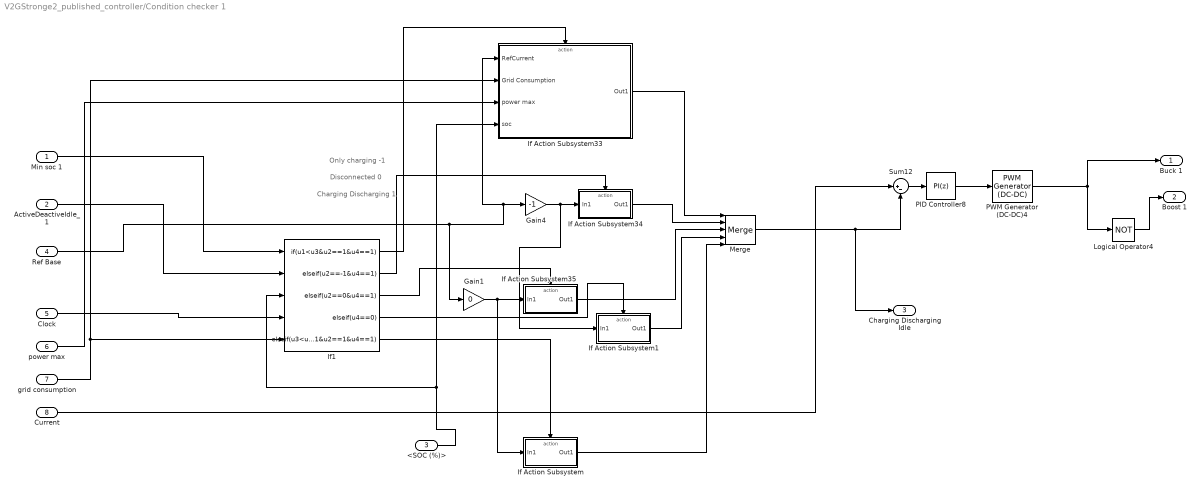
== system V2GStronge2_published_controller/Condition checker 1 ==
  note: Charging Discharging 1
  note: Disconnected 0
  note: Only charging -1
  Min soc 1 : Inport
  ActiveDeactiveIdle_1 : Inport  Port=2
  <SOC (%)> : Inport  Port=3
  Ref Base : Inport  Port=4
  Clock : Inport  Port=5
  power max : Inport  Port=6
  grid consumption : Inport  Port=7
  Current : Inport  Port=8
  Gain1 : Gain  Gain=0
  Gain4 : Gain  Gain=-1
  If Action Subsystem : Subsystem  TreatAsAtomicUnit=on
  If Action Subsystem1 : Subsystem  TreatAsAtomicUnit=on
  If Action Subsystem33 : Subsystem  TreatAsAtomicUnit=on
  If Action Subsystem34 : Subsystem  TreatAsAtomicUnit=on
  If Action Subsystem35 : Subsystem  TreatAsAtomicUnit=on
  If1 : If  NumInputs=5  IfExpression=u1<u3&u2==1&u4==1  ElseIfExpressions=u2==-1&u4==1,u2==0&u4==1,u4==0,u3<u1&u2==1&u4==1  ShowElse=off
  Logical Operator4 : Logic  Operator=NOT  AllPortsSameDT=off  OutDataTypeStr=boolean
  Merge : Merge  Inputs=5
  PID Controller8 : slpidlib/PID Controller  Controller=PI  Form=Parallel  TimeDomain=Discrete-time  UseExternalTs=off  SampleTime=-1  IntegratorMethod=Forward Euler  FilterMethod=Forward Euler  ControllerParametersSource=internal  P=0.005  I=10  UseKiTs=off  D=0  UseExternalDerivativeSource=off  N=100  UseFilter=on  TunerSelectOption=Transfer Function Based (PID Tuner App)  InitialConditionSource=internal  InitialConditionForIntegrator=0  InitialConditionForFilter=0  DifferentiatorICPrevScaledInput=0  ExternalReset=none  TrackingMode=off  Kt=1  LimitOutput=on  SatLimitsSource=internal  UpperSaturationLimit=0.95  LowerSaturationLimit=0  LinearizeAsGain=on  AntiWindupMode=none  Kb=1  LimitIntegrator=off  UpperIntegratorSaturationLimit=inf  LowerIntegratorSaturationLimit=-inf  POutMin=[]  POutMax=[]  IOutMin=[]  IOutMax=[]  DOutMin=[]  DOutMax=[]  NOutMin=[]  NOutMax=[]  SumOutMin=[]  SumOutMax=[]  SaturationOutMin=[]  SaturationOutMax=[]  PParamMin=[]  PParamMax=[]  IParamMin=[]  IParamMax=[]  DParamMin=[]  DParamMax=[]  NParamMin=[]  NParamMax=[]  KbParamMin=[]  KbParamMax=[]  KtParamMin=[]  KtParamMax=[]  KbOutMin=[]  KbOutMax=[]  KtOutMin=[]  KtOutMax=[]  IntegratorOutMin=[]  IntegratorOutMax=[]  FilterOutMin=[]  FilterOutMax=[]  SumI1OutMin=[]  SumI1OutMax=[]  SumI2OutMin=[]  SumI2OutMax=[]  SumI3OutMin=[]  SumI3OutMax=[]  SumI4OutMin=[]  SumI4OutMax=[]  SumDOutMin=[]  SumDOutMax=[]  DifferentiatorOutMin=[]  DifferentiatorOutMax=[]  FilterDiffOutCoefMin=[]  FilterDiffOutCoefMax=[]  ReciprocalOutMin=[]  ReciprocalOutMax=[]  SumDenOutMin=[]  SumDenOutMax=[]  SumNumOutMin=[]  SumNumOutMax=[]  DivideOutMin=[]  DivideOutMax=[]  UdiffTsProdOutMin=[]  UdiffTsProdOutMax=[]  NTsProdOutMin=[]  NTsProdOutMax=[]  UintegralTsProdOutMin=[]  UintegralTsProdOutMax=[]  UngainTsProdOutMin=[]  UngainTsProdOutMax=[]  ClampingZeroOutDataTypeStr=Inherit: Inherit via back propagation  ClampingZeroOutMin=[]  ClampingZeroOutMax=[]  FilterDenConstantOutDataTypeStr=Inherit: Inherit via back propagation  FilterDenConstantOutMin=[]  FilterDenConstantOutMax=[]  PCopyOutDataTypeStr=Inherit: Inherit via back propagation  PCopyOutMin=[]  PCopyOutMax=[]  NCopyOutDataTypeStr=Inherit: Inherit via back propagation  NCopyOutMin=[]  NCopyOutMax=[]  IntegratorContinuousStateAttributes=''  IntegratorStateMustResolveToSignalObject=off  IntegratorRTWStateStorageClass=Auto  FilterContinuousStateAttributes=''  FilterStateMustResolveToSignalObject=off  FilterRTWStateStorageClass=Auto  ParallelPVariant=InternalParameters  IdealPVariant=Disabled  IVariant=InternalParameters  DVariant=Disabled  IntegratorVariant=Discrete  SatVariant=Enabled  AWVariant=Passthrough  PCopyVariant=Disabled  TRVariant=Disabled  FdbkBlocksVariant=Forward  IdealPFdbkVariant=Disabled  SatFdbkVariant=Disabled  DerivativeFilterVariant=Disabled  NVariant=Disabled  NCopyVariant=Disabled_SignalSpec  FilterICVariant=Disabled  IntegratorICVariant=InternalICs  ExternalResetVariant=Disabled  TRSumVariant=Passthrough  SumFdbkVariant=Disabled  SumVariant=Sum_PI  TsampFilterVariant=InternalTs  TsampNgainVariant=Passthrough  TsampIntegralVariant=Disabled_SignalSpec  ExternalSaturationOutDataTypeStr=Inherit: Same as second input  DerivativeSourceVariant=Disabled
  PWM Generator (DC-DC)4 : spsPWMGeneratorDCDCLib/PWM Generator (DC-DC)  Fsw=60  Ts=0
  Sum12 : Sum  Inputs=|+-
  Buck 1 : Outport
  Boost 1 : Outport  Port=2
  Charging Discharging Idle : Outport  Port=3
  wires:
  Current/1 -> Sum12/1
  Sum12/1 -> PID Controller8/1
  If1/3 -> If Action Subsystem35/Action
  PID Controller8/1 -> PWM Generator (DC-DC)4/1
  If1/1 -> If Action Subsystem33/Action
  If Action Subsystem35/1(Out1) -> Merge/3
  Min soc 1/1 -> If1/1
  Logical Operator4/1 -> Boost 1/1
  Ref Base/1 -> If Action Subsystem33/1(RefCurrent), Gain4/1, Gain1/1
  If Action Subsystem33/1(Out1) -> Merge/1
  Gain4/1 -> If Action Subsystem1/1(In1), If Action Subsystem34/1(In1)
  ActiveDeactiveIdle_1/1 -> If1/2
  PWM Generator (DC-DC)4/1 -> Buck 1/1, Logical Operator4/1
  If Action Subsystem34/1(Out1) -> Merge/2
  Merge/1 -> Charging Discharging Idle/1, Sum12/2
  If1/2 -> If Action Subsystem34/Action
  <SOC (%)>/1 -> If1/3, If Action Subsystem33/4(soc)
  Clock/1 -> If1/4
  If Action Subsystem1/1(Out1) -> Merge/4
  If1/4 -> If Action Subsystem1/Action
  grid consumption/1 -> If1/5, If Action Subsystem33/2(Grid Consumption)
  power max/1 -> If Action Subsystem33/3(power max)
  Gain1/1 -> If Action Subsystem/1(In1), If Action Subsystem35/1(In1)
  If1/5 -> If Action Subsystem/Action
  If Action Subsystem/1(Out1) -> Merge/5
